simulink model "gol_cell_cl"  (R2022a)
settings: Solver=VariableStepAuto  StartTime=0.0  StopTime=10.0  RelTol=1e-3
libraries: simulink_extras x9
settings Model: Creator=SoLoMoN  LastModifiedBy=SoLoMoN

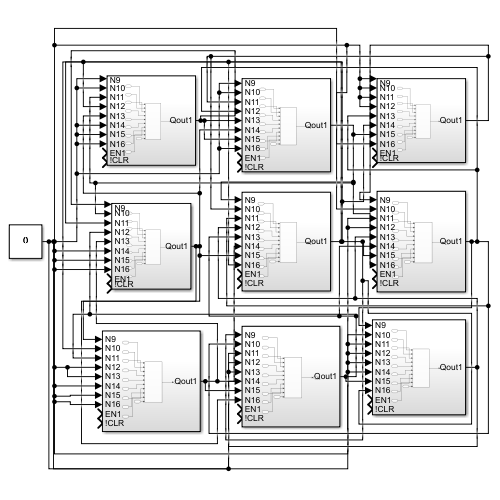
[thumbnail: Simulink's stored preview of the top-level diagram]
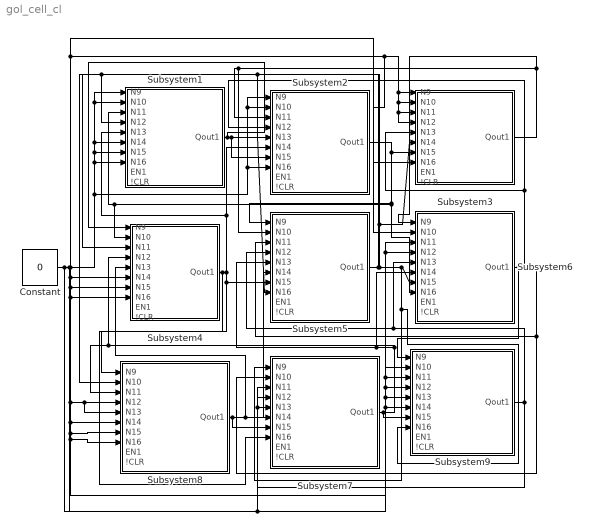
== system gol_cell_cl ==
  Constant : Constant  Value=0
  Subsystem1 : Subsystem
  Subsystem2 : Subsystem
  Subsystem3 : Subsystem
  Subsystem4 : Subsystem
  Subsystem5 : Subsystem
  Subsystem6 : Subsystem
  Subsystem7 : Subsystem
  Subsystem8 : Subsystem
  Subsystem9 : Subsystem
  wires:
  Subsystem4/1(Qout1) -> Subsystem7/8(N16), Subsystem8/1(N9), Subsystem5/7(N15), Subsystem1/5(N13), Subsystem2/6(N14)
  Subsystem2/1(Qout1) -> Subsystem6/8(N16), Subsystem4/2(N10), Subsystem1/3(N11), Subsystem5/1(N9), Subsystem3/7(N15)
  Subsystem3/1(Qout1) -> Subsystem6/1(N9), Subsystem2/3(N11), Subsystem5/2(N10)
  Subsystem6/1(Qout1) -> Subsystem7/2(N10), Subsystem5/3(N11), Subsystem3/5(N13), Subsystem2/4(N12), Subsystem9/1(N9)
  Subsystem9/1(Qout1) -> Subsystem7/3(N11), Subsystem6/5(N13), Subsystem5/4(N12)
  Subsystem7/1(Qout1) -> Subsystem9/7(N15), Subsystem8/3(N11), Subsystem4/4(N12), Subsystem6/6(N14), Subsystem5/5(N13)
  Subsystem8/1(Qout1) -> Subsystem7/7(N15), Subsystem4/5(N13), Subsystem5/6(N14)
  Subsystem1/1(Qout1) -> Subsystem4/1(N9), Subsystem2/7(N15), Subsystem5/8(N16)
  Constant/1 -> Subsystem9/6(N14), Subsystem9/3(N11), Subsystem9/2(N10), Subsystem9/4(N12), Subsystem9/5(N13), Subsystem7/6(N14), Subsystem7/5(N13), Subsystem7/4(N12), Subsystem6/2(N10), Subsystem3/4(N12), Subsystem3/3(N11), Subsystem3/2(N10), Subsystem3/1(N9), Subsystem3/8(N16), Subsystem8/5(N13), Subsystem8/4(N12), Subsystem8/6(N14), Subsystem8/7(N15), Subsystem8/8(N16), Subsystem6/4(N12), Subsystem6/3(N11), Subsystem4/8(N16), Subsystem4/7(N15), Subsystem4/6(N14), Subsystem1/7(N15), Subsystem1/6(N14), Subsystem1/2(N10), Subsystem1/1(N9), Subsystem1/8(N16), Subsystem2/8(N16), Subsystem2/2(N10), Subsystem2/1(N9)
  Subsystem5/1(Qout1) -> Subsystem9/8(N16), Subsystem7/1(N9), Subsystem6/7(N15), Subsystem4/3(N11), Subsystem1/4(N12), Subsystem2/5(N13), Subsystem3/6(N14), Subsystem8/2(N10)

== system gol_cell_cl/Subsystem1 ==
  N9 : Inport
  N10 : Inport  Port=2
  N11 : Inport  Port=3
  N12 : Inport  Port=4
  N13 : Inport  Port=5
  N14 : Inport  Port=6
  N15 : Inport  Port=7
  N16 : Inport  Port=8
  EN1 : Inport  Port=9
  !CLR : Inport  Port=10
  cell (1,1) : Subsystem
  Qout1 : Outport
  wires:
  EN1/1 -> cell (1,1)/8(EN)
  N12/1 -> cell (1,1)/4(N4)
  N13/1 -> cell (1,1)/5(N5)
  N14/1 -> cell (1,1)/6(N6)
  N15/1 -> cell (1,1)/7(N7)
  N10/1 -> cell (1,1)/2(N2)
  cell (1,1)/1(Qout) -> Qout1/1
  !CLR/1 -> cell (1,1)/10(!CLR)
  N9/1 -> cell (1,1)/1(N1)
  N11/1 -> cell (1,1)/3(N3)
  N16/1 -> cell (1,1)/9(N8)

== system gol_cell_cl/Subsystem2 ==
  N9 : Inport
  N10 : Inport  Port=2
  N11 : Inport  Port=3
  N12 : Inport  Port=4
  N13 : Inport  Port=5
  N14 : Inport  Port=6
  N15 : Inport  Port=7
  N16 : Inport  Port=8
  EN1 : Inport  Port=9
  !CLR : Inport  Port=10
  cell (1,1) : Subsystem
  Qout1 : Outport
  wires:
  EN1/1 -> cell (1,1)/8(EN)
  N12/1 -> cell (1,1)/4(N4)
  N13/1 -> cell (1,1)/5(N5)
  N14/1 -> cell (1,1)/6(N6)
  N15/1 -> cell (1,1)/7(N7)
  N10/1 -> cell (1,1)/2(N2)
  cell (1,1)/1(Qout) -> Qout1/1
  !CLR/1 -> cell (1,1)/10(!CLR)
  N9/1 -> cell (1,1)/1(N1)
  N11/1 -> cell (1,1)/3(N3)
  N16/1 -> cell (1,1)/9(N8)

== system gol_cell_cl/Subsystem3 ==
  N9 : Inport
  N10 : Inport  Port=2
  N11 : Inport  Port=3
  N12 : Inport  Port=4
  N13 : Inport  Port=5
  N14 : Inport  Port=6
  N15 : Inport  Port=7
  N16 : Inport  Port=8
  EN1 : Inport  Port=9
  !CLR : Inport  Port=10
  cell (1,1) : Subsystem
  Qout1 : Outport
  wires:
  EN1/1 -> cell (1,1)/8(EN)
  N12/1 -> cell (1,1)/4(N4)
  N13/1 -> cell (1,1)/5(N5)
  N14/1 -> cell (1,1)/6(N6)
  N15/1 -> cell (1,1)/7(N7)
  N10/1 -> cell (1,1)/2(N2)
  cell (1,1)/1(Qout) -> Qout1/1
  !CLR/1 -> cell (1,1)/10(!CLR)
  N9/1 -> cell (1,1)/1(N1)
  N11/1 -> cell (1,1)/3(N3)
  N16/1 -> cell (1,1)/9(N8)

== system gol_cell_cl/Subsystem4 ==
  N9 : Inport
  N10 : Inport  Port=2
  N11 : Inport  Port=3
  N12 : Inport  Port=4
  N13 : Inport  Port=5
  N14 : Inport  Port=6
  N15 : Inport  Port=7
  N16 : Inport  Port=8
  EN1 : Inport  Port=9
  !CLR : Inport  Port=10
  cell (1,1) : Subsystem
  Qout1 : Outport
  wires:
  EN1/1 -> cell (1,1)/8(EN)
  N12/1 -> cell (1,1)/4(N4)
  N13/1 -> cell (1,1)/5(N5)
  N14/1 -> cell (1,1)/6(N6)
  N15/1 -> cell (1,1)/7(N7)
  N10/1 -> cell (1,1)/2(N2)
  cell (1,1)/1(Qout) -> Qout1/1
  !CLR/1 -> cell (1,1)/10(!CLR)
  N9/1 -> cell (1,1)/1(N1)
  N11/1 -> cell (1,1)/3(N3)
  N16/1 -> cell (1,1)/9(N8)

== system gol_cell_cl/Subsystem5 ==
  N9 : Inport
  N10 : Inport  Port=2
  N11 : Inport  Port=3
  N12 : Inport  Port=4
  N13 : Inport  Port=5
  N14 : Inport  Port=6
  N15 : Inport  Port=7
  N16 : Inport  Port=8
  EN1 : Inport  Port=9
  !CLR : Inport  Port=10
  cell (1,1) : Subsystem
  Qout1 : Outport
  wires:
  EN1/1 -> cell (1,1)/8(EN)
  N12/1 -> cell (1,1)/4(N4)
  N13/1 -> cell (1,1)/5(N5)
  N14/1 -> cell (1,1)/6(N6)
  N15/1 -> cell (1,1)/7(N7)
  N10/1 -> cell (1,1)/2(N2)
  cell (1,1)/1(Qout) -> Qout1/1
  !CLR/1 -> cell (1,1)/10(!CLR)
  N9/1 -> cell (1,1)/1(N1)
  N11/1 -> cell (1,1)/3(N3)
  N16/1 -> cell (1,1)/9(N8)

== system gol_cell_cl/Subsystem6 ==
  N9 : Inport
  N10 : Inport  Port=2
  N11 : Inport  Port=3
  N12 : Inport  Port=4
  N13 : Inport  Port=5
  N14 : Inport  Port=6
  N15 : Inport  Port=7
  N16 : Inport  Port=8
  EN1 : Inport  Port=9
  !CLR : Inport  Port=10
  cell (1,1) : Subsystem
  Qout1 : Outport
  wires:
  EN1/1 -> cell (1,1)/8(EN)
  N12/1 -> cell (1,1)/4(N4)
  N13/1 -> cell (1,1)/5(N5)
  N14/1 -> cell (1,1)/6(N6)
  N15/1 -> cell (1,1)/7(N7)
  N10/1 -> cell (1,1)/2(N2)
  cell (1,1)/1(Qout) -> Qout1/1
  !CLR/1 -> cell (1,1)/10(!CLR)
  N9/1 -> cell (1,1)/1(N1)
  N11/1 -> cell (1,1)/3(N3)
  N16/1 -> cell (1,1)/9(N8)

== system gol_cell_cl/Subsystem7 ==
  N9 : Inport
  N10 : Inport  Port=2
  N11 : Inport  Port=3
  N12 : Inport  Port=4
  N13 : Inport  Port=5
  N14 : Inport  Port=6
  N15 : Inport  Port=7
  N16 : Inport  Port=8
  EN1 : Inport  Port=9
  !CLR : Inport  Port=10
  cell (1,1) : Subsystem
  Qout1 : Outport
  wires:
  EN1/1 -> cell (1,1)/8(EN)
  N12/1 -> cell (1,1)/4(N4)
  N13/1 -> cell (1,1)/5(N5)
  N14/1 -> cell (1,1)/6(N6)
  N15/1 -> cell (1,1)/7(N7)
  N10/1 -> cell (1,1)/2(N2)
  cell (1,1)/1(Qout) -> Qout1/1
  !CLR/1 -> cell (1,1)/10(!CLR)
  N9/1 -> cell (1,1)/1(N1)
  N11/1 -> cell (1,1)/3(N3)
  N16/1 -> cell (1,1)/9(N8)

== system gol_cell_cl/Subsystem8 ==
  N9 : Inport
  N10 : Inport  Port=2
  N11 : Inport  Port=3
  N12 : Inport  Port=4
  N13 : Inport  Port=5
  N14 : Inport  Port=6
  N15 : Inport  Port=7
  N16 : Inport  Port=8
  EN1 : Inport  Port=9
  !CLR : Inport  Port=10
  cell (1,1) : Subsystem
  Qout1 : Outport
  wires:
  EN1/1 -> cell (1,1)/8(EN)
  N12/1 -> cell (1,1)/4(N4)
  N13/1 -> cell (1,1)/5(N5)
  N14/1 -> cell (1,1)/6(N6)
  N15/1 -> cell (1,1)/7(N7)
  N10/1 -> cell (1,1)/2(N2)
  cell (1,1)/1(Qout) -> Qout1/1
  !CLR/1 -> cell (1,1)/10(!CLR)
  N9/1 -> cell (1,1)/1(N1)
  N11/1 -> cell (1,1)/3(N3)
  N16/1 -> cell (1,1)/9(N8)

== system gol_cell_cl/Subsystem9 ==
  N9 : Inport
  N10 : Inport  Port=2
  N11 : Inport  Port=3
  N12 : Inport  Port=4
  N13 : Inport  Port=5
  N14 : Inport  Port=6
  N15 : Inport  Port=7
  N16 : Inport  Port=8
  EN1 : Inport  Port=9
  !CLR : Inport  Port=10
  cell (1,1) : Subsystem
  Qout1 : Outport
  wires:
  EN1/1 -> cell (1,1)/8(EN)
  N12/1 -> cell (1,1)/4(N4)
  N13/1 -> cell (1,1)/5(N5)
  N14/1 -> cell (1,1)/6(N6)
  N15/1 -> cell (1,1)/7(N7)
  N10/1 -> cell (1,1)/2(N2)
  cell (1,1)/1(Qout) -> Qout1/1
  !CLR/1 -> cell (1,1)/10(!CLR)
  N9/1 -> cell (1,1)/1(N1)
  N11/1 -> cell (1,1)/3(N3)
  N16/1 -> cell (1,1)/9(N8)

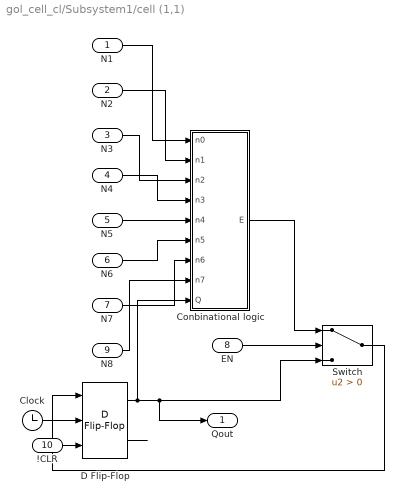
== system gol_cell_cl/Subsystem1/cell (1,1) ==
  N1 : Inport
  N2 : Inport  Port=2
  N3 : Inport  Port=3
  N4 : Inport  Port=4
  N5 : Inport  Port=5
  N6 : Inport  Port=6
  N7 : Inport  Port=7
  EN : Inport  Port=8
  N8 : Inport  Port=9
  !CLR : Inport  Port=10
  Clock : Clock
  Conbinational logic : Subsystem
  D Flip-Flop : simulink_extras/Flip Flops/D Flip-Flop
  Switch : Switch  Criteria=u2 > Threshold  SaturateOnIntegerOverflow=off  InputSameDT=off
  Qout : Outport
  wires:
  N3/1 -> Conbinational logic/3(n2)
  N1/1 -> Conbinational logic/1(n0)
  Clock/1 -> D Flip-Flop/2
  Conbinational logic/1(E) -> Switch/1
  Switch/1 -> D Flip-Flop/1
  D Flip-Flop/1 -> Qout/1, Switch/3, Conbinational logic/9(Q)
  N6/1 -> Conbinational logic/6(n5)
  EN/1 -> Switch/2
  N2/1 -> Conbinational logic/2(n1)
  N7/1 -> Conbinational logic/7(n6)
  N4/1 -> Conbinational logic/4(n3)
  N5/1 -> Conbinational logic/5(n4)
  N8/1 -> Conbinational logic/8(n7)
  !CLR/1 -> D Flip-Flop/3
  D Flip-Flop/2 -> ?

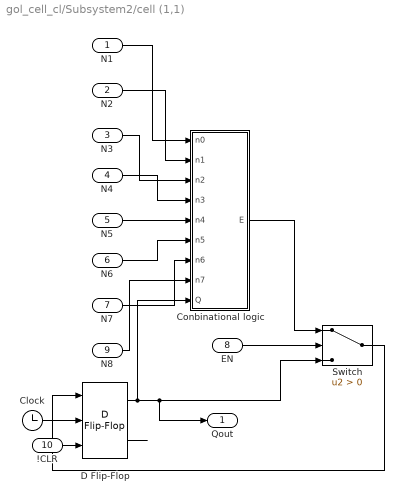
== system gol_cell_cl/Subsystem2/cell (1,1) ==
  N1 : Inport
  N2 : Inport  Port=2
  N3 : Inport  Port=3
  N4 : Inport  Port=4
  N5 : Inport  Port=5
  N6 : Inport  Port=6
  N7 : Inport  Port=7
  EN : Inport  Port=8
  N8 : Inport  Port=9
  !CLR : Inport  Port=10
  Clock : Clock
  Conbinational logic : Subsystem
  D Flip-Flop : simulink_extras/Flip Flops/D Flip-Flop
  Switch : Switch  Criteria=u2 > Threshold  SaturateOnIntegerOverflow=off  InputSameDT=off
  Qout : Outport
  wires:
  N3/1 -> Conbinational logic/3(n2)
  N1/1 -> Conbinational logic/1(n0)
  Clock/1 -> D Flip-Flop/2
  Conbinational logic/1(E) -> Switch/1
  Switch/1 -> D Flip-Flop/1
  D Flip-Flop/1 -> Qout/1, Switch/3, Conbinational logic/9(Q)
  N6/1 -> Conbinational logic/6(n5)
  EN/1 -> Switch/2
  N2/1 -> Conbinational logic/2(n1)
  N7/1 -> Conbinational logic/7(n6)
  N4/1 -> Conbinational logic/4(n3)
  N5/1 -> Conbinational logic/5(n4)
  N8/1 -> Conbinational logic/8(n7)
  !CLR/1 -> D Flip-Flop/3
  D Flip-Flop/2 -> ?

== system gol_cell_cl/Subsystem3/cell (1,1) ==
  N1 : Inport
  N2 : Inport  Port=2
  N3 : Inport  Port=3
  N4 : Inport  Port=4
  N5 : Inport  Port=5
  N6 : Inport  Port=6
  N7 : Inport  Port=7
  EN : Inport  Port=8
  N8 : Inport  Port=9
  !CLR : Inport  Port=10
  Clock : Clock
  Conbinational logic : Subsystem
  D Flip-Flop : simulink_extras/Flip Flops/D Flip-Flop
  Switch : Switch  Criteria=u2 > Threshold  SaturateOnIntegerOverflow=off  InputSameDT=off
  Qout : Outport
  wires:
  N3/1 -> Conbinational logic/3(n2)
  N1/1 -> Conbinational logic/1(n0)
  Clock/1 -> D Flip-Flop/2
  Conbinational logic/1(E) -> Switch/1
  Switch/1 -> D Flip-Flop/1
  D Flip-Flop/1 -> Qout/1, Switch/3, Conbinational logic/9(Q)
  N6/1 -> Conbinational logic/6(n5)
  EN/1 -> Switch/2
  N2/1 -> Conbinational logic/2(n1)
  N7/1 -> Conbinational logic/7(n6)
  N4/1 -> Conbinational logic/4(n3)
  N5/1 -> Conbinational logic/5(n4)
  N8/1 -> Conbinational logic/8(n7)
  !CLR/1 -> D Flip-Flop/3
  D Flip-Flop/2 -> ?

== system gol_cell_cl/Subsystem4/cell (1,1) ==
  N1 : Inport
  N2 : Inport  Port=2
  N3 : Inport  Port=3
  N4 : Inport  Port=4
  N5 : Inport  Port=5
  N6 : Inport  Port=6
  N7 : Inport  Port=7
  EN : Inport  Port=8
  N8 : Inport  Port=9
  !CLR : Inport  Port=10
  Clock : Clock
  Conbinational logic : Subsystem
  D Flip-Flop : simulink_extras/Flip Flops/D Flip-Flop
  Switch : Switch  Criteria=u2 > Threshold  SaturateOnIntegerOverflow=off  InputSameDT=off
  Qout : Outport
  wires:
  N3/1 -> Conbinational logic/3(n2)
  N1/1 -> Conbinational logic/1(n0)
  Clock/1 -> D Flip-Flop/2
  Conbinational logic/1(E) -> Switch/1
  Switch/1 -> D Flip-Flop/1
  D Flip-Flop/1 -> Qout/1, Switch/3, Conbinational logic/9(Q)
  N6/1 -> Conbinational logic/6(n5)
  EN/1 -> Switch/2
  N2/1 -> Conbinational logic/2(n1)
  N7/1 -> Conbinational logic/7(n6)
  N4/1 -> Conbinational logic/4(n3)
  N5/1 -> Conbinational logic/5(n4)
  N8/1 -> Conbinational logic/8(n7)
  !CLR/1 -> D Flip-Flop/3
  D Flip-Flop/2 -> ?

== system gol_cell_cl/Subsystem5/cell (1,1) ==
  N1 : Inport
  N2 : Inport  Port=2
  N3 : Inport  Port=3
  N4 : Inport  Port=4
  N5 : Inport  Port=5
  N6 : Inport  Port=6
  N7 : Inport  Port=7
  EN : Inport  Port=8
  N8 : Inport  Port=9
  !CLR : Inport  Port=10
  Clock : Clock
  Conbinational logic : Subsystem
  D Flip-Flop : simulink_extras/Flip Flops/D Flip-Flop
  Switch : Switch  Criteria=u2 > Threshold  SaturateOnIntegerOverflow=off  InputSameDT=off
  Qout : Outport
  wires:
  N3/1 -> Conbinational logic/3(n2)
  N1/1 -> Conbinational logic/1(n0)
  Clock/1 -> D Flip-Flop/2
  Conbinational logic/1(E) -> Switch/1
  Switch/1 -> D Flip-Flop/1
  D Flip-Flop/1 -> Qout/1, Switch/3, Conbinational logic/9(Q)
  N6/1 -> Conbinational logic/6(n5)
  EN/1 -> Switch/2
  N2/1 -> Conbinational logic/2(n1)
  N7/1 -> Conbinational logic/7(n6)
  N4/1 -> Conbinational logic/4(n3)
  N5/1 -> Conbinational logic/5(n4)
  N8/1 -> Conbinational logic/8(n7)
  !CLR/1 -> D Flip-Flop/3
  D Flip-Flop/2 -> ?

== system gol_cell_cl/Subsystem6/cell (1,1) ==
  N1 : Inport
  N2 : Inport  Port=2
  N3 : Inport  Port=3
  N4 : Inport  Port=4
  N5 : Inport  Port=5
  N6 : Inport  Port=6
  N7 : Inport  Port=7
  EN : Inport  Port=8
  N8 : Inport  Port=9
  !CLR : Inport  Port=10
  Clock : Clock
  Conbinational logic : Subsystem
  D Flip-Flop : simulink_extras/Flip Flops/D Flip-Flop
  Switch : Switch  Criteria=u2 > Threshold  SaturateOnIntegerOverflow=off  InputSameDT=off
  Qout : Outport
  wires:
  N3/1 -> Conbinational logic/3(n2)
  N1/1 -> Conbinational logic/1(n0)
  Clock/1 -> D Flip-Flop/2
  Conbinational logic/1(E) -> Switch/1
  Switch/1 -> D Flip-Flop/1
  D Flip-Flop/1 -> Qout/1, Switch/3, Conbinational logic/9(Q)
  N6/1 -> Conbinational logic/6(n5)
  EN/1 -> Switch/2
  N2/1 -> Conbinational logic/2(n1)
  N7/1 -> Conbinational logic/7(n6)
  N4/1 -> Conbinational logic/4(n3)
  N5/1 -> Conbinational logic/5(n4)
  N8/1 -> Conbinational logic/8(n7)
  !CLR/1 -> D Flip-Flop/3
  D Flip-Flop/2 -> ?

== system gol_cell_cl/Subsystem7/cell (1,1) ==
  N1 : Inport
  N2 : Inport  Port=2
  N3 : Inport  Port=3
  N4 : Inport  Port=4
  N5 : Inport  Port=5
  N6 : Inport  Port=6
  N7 : Inport  Port=7
  EN : Inport  Port=8
  N8 : Inport  Port=9
  !CLR : Inport  Port=10
  Clock : Clock
  Conbinational logic : Subsystem
  D Flip-Flop : simulink_extras/Flip Flops/D Flip-Flop
  Switch : Switch  Criteria=u2 > Threshold  SaturateOnIntegerOverflow=off  InputSameDT=off
  Qout : Outport
  wires:
  N3/1 -> Conbinational logic/3(n2)
  N1/1 -> Conbinational logic/1(n0)
  Clock/1 -> D Flip-Flop/2
  Conbinational logic/1(E) -> Switch/1
  Switch/1 -> D Flip-Flop/1
  D Flip-Flop/1 -> Qout/1, Switch/3, Conbinational logic/9(Q)
  N6/1 -> Conbinational logic/6(n5)
  EN/1 -> Switch/2
  N2/1 -> Conbinational logic/2(n1)
  N7/1 -> Conbinational logic/7(n6)
  N4/1 -> Conbinational logic/4(n3)
  N5/1 -> Conbinational logic/5(n4)
  N8/1 -> Conbinational logic/8(n7)
  !CLR/1 -> D Flip-Flop/3
  D Flip-Flop/2 -> ?

== system gol_cell_cl/Subsystem8/cell (1,1) ==
  N1 : Inport
  N2 : Inport  Port=2
  N3 : Inport  Port=3
  N4 : Inport  Port=4
  N5 : Inport  Port=5
  N6 : Inport  Port=6
  N7 : Inport  Port=7
  EN : Inport  Port=8
  N8 : Inport  Port=9
  !CLR : Inport  Port=10
  Clock : Clock
  Conbinational logic : Subsystem
  D Flip-Flop : simulink_extras/Flip Flops/D Flip-Flop
  Switch : Switch  Criteria=u2 > Threshold  SaturateOnIntegerOverflow=off  InputSameDT=off
  Qout : Outport
  wires:
  N3/1 -> Conbinational logic/3(n2)
  N1/1 -> Conbinational logic/1(n0)
  Clock/1 -> D Flip-Flop/2
  Conbinational logic/1(E) -> Switch/1
  Switch/1 -> D Flip-Flop/1
  D Flip-Flop/1 -> Qout/1, Switch/3, Conbinational logic/9(Q)
  N6/1 -> Conbinational logic/6(n5)
  EN/1 -> Switch/2
  N2/1 -> Conbinational logic/2(n1)
  N7/1 -> Conbinational logic/7(n6)
  N4/1 -> Conbinational logic/4(n3)
  N5/1 -> Conbinational logic/5(n4)
  N8/1 -> Conbinational logic/8(n7)
  !CLR/1 -> D Flip-Flop/3
  D Flip-Flop/2 -> ?

== system gol_cell_cl/Subsystem9/cell (1,1) ==
  N1 : Inport
  N2 : Inport  Port=2
  N3 : Inport  Port=3
  N4 : Inport  Port=4
  N5 : Inport  Port=5
  N6 : Inport  Port=6
  N7 : Inport  Port=7
  EN : Inport  Port=8
  N8 : Inport  Port=9
  !CLR : Inport  Port=10
  Clock : Clock
  Conbinational logic : Subsystem
  D Flip-Flop : simulink_extras/Flip Flops/D Flip-Flop
  Switch : Switch  Criteria=u2 > Threshold  SaturateOnIntegerOverflow=off  InputSameDT=off
  Qout : Outport
  wires:
  N3/1 -> Conbinational logic/3(n2)
  N1/1 -> Conbinational logic/1(n0)
  Clock/1 -> D Flip-Flop/2
  Conbinational logic/1(E) -> Switch/1
  Switch/1 -> D Flip-Flop/1
  D Flip-Flop/1 -> Qout/1, Switch/3, Conbinational logic/9(Q)
  N6/1 -> Conbinational logic/6(n5)
  EN/1 -> Switch/2
  N2/1 -> Conbinational logic/2(n1)
  N7/1 -> Conbinational logic/7(n6)
  N4/1 -> Conbinational logic/4(n3)
  N5/1 -> Conbinational logic/5(n4)
  N8/1 -> Conbinational logic/8(n7)
  !CLR/1 -> D Flip-Flop/3
  D Flip-Flop/2 -> ?

== system gol_cell_cl/Subsystem1/cell (1,1)/Conbinational logic ==
  n0 : Inport
  n1 : Inport  Port=2
  n2 : Inport  Port=3
  n3 : Inport  Port=4
  n4 : Inport  Port=5
  n5 : Inport  Port=6
  n6 : Inport  Port=7
  n7 : Inport  Port=8
  Q : Inport  Port=9
  PACK : Subsystem
  E : Outport
  wires:
  n0/1 -> PACK/1(n0)
  n1/1 -> PACK/2(n1)
  n2/1 -> PACK/3(n2)
  n3/1 -> PACK/4(n3)
  n4/1 -> PACK/5(n4)
  n5/1 -> PACK/6(n5)
  n6/1 -> PACK/7(n6)
  n7/1 -> PACK/8(n7)
  Q/1 -> PACK/9(Q)
  PACK/1(E) -> E/1

== system gol_cell_cl/Subsystem2/cell (1,1)/Conbinational logic ==
  n0 : Inport
  n1 : Inport  Port=2
  n2 : Inport  Port=3
  n3 : Inport  Port=4
  n4 : Inport  Port=5
  n5 : Inport  Port=6
  n6 : Inport  Port=7
  n7 : Inport  Port=8
  Q : Inport  Port=9
  PACK : Subsystem
  E : Outport
  wires:
  n0/1 -> PACK/1(n0)
  n1/1 -> PACK/2(n1)
  n2/1 -> PACK/3(n2)
  n3/1 -> PACK/4(n3)
  n4/1 -> PACK/5(n4)
  n5/1 -> PACK/6(n5)
  n6/1 -> PACK/7(n6)
  n7/1 -> PACK/8(n7)
  Q/1 -> PACK/9(Q)
  PACK/1(E) -> E/1

== system gol_cell_cl/Subsystem3/cell (1,1)/Conbinational logic ==
  n0 : Inport
  n1 : Inport  Port=2
  n2 : Inport  Port=3
  n3 : Inport  Port=4
  n4 : Inport  Port=5
  n5 : Inport  Port=6
  n6 : Inport  Port=7
  n7 : Inport  Port=8
  Q : Inport  Port=9
  PACK : Subsystem
  E : Outport
  wires:
  n0/1 -> PACK/1(n0)
  n1/1 -> PACK/2(n1)
  n2/1 -> PACK/3(n2)
  n3/1 -> PACK/4(n3)
  n4/1 -> PACK/5(n4)
  n5/1 -> PACK/6(n5)
  n6/1 -> PACK/7(n6)
  n7/1 -> PACK/8(n7)
  Q/1 -> PACK/9(Q)
  PACK/1(E) -> E/1

== system gol_cell_cl/Subsystem4/cell (1,1)/Conbinational logic ==
  n0 : Inport
  n1 : Inport  Port=2
  n2 : Inport  Port=3
  n3 : Inport  Port=4
  n4 : Inport  Port=5
  n5 : Inport  Port=6
  n6 : Inport  Port=7
  n7 : Inport  Port=8
  Q : Inport  Port=9
  PACK : Subsystem
  E : Outport
  wires:
  n0/1 -> PACK/1(n0)
  n1/1 -> PACK/2(n1)
  n2/1 -> PACK/3(n2)
  n3/1 -> PACK/4(n3)
  n4/1 -> PACK/5(n4)
  n5/1 -> PACK/6(n5)
  n6/1 -> PACK/7(n6)
  n7/1 -> PACK/8(n7)
  Q/1 -> PACK/9(Q)
  PACK/1(E) -> E/1

== system gol_cell_cl/Subsystem5/cell (1,1)/Conbinational logic ==
  n0 : Inport
  n1 : Inport  Port=2
  n2 : Inport  Port=3
  n3 : Inport  Port=4
  n4 : Inport  Port=5
  n5 : Inport  Port=6
  n6 : Inport  Port=7
  n7 : Inport  Port=8
  Q : Inport  Port=9
  PACK : Subsystem
  E : Outport
  wires:
  n0/1 -> PACK/1(n0)
  n1/1 -> PACK/2(n1)
  n2/1 -> PACK/3(n2)
  n3/1 -> PACK/4(n3)
  n4/1 -> PACK/5(n4)
  n5/1 -> PACK/6(n5)
  n6/1 -> PACK/7(n6)
  n7/1 -> PACK/8(n7)
  Q/1 -> PACK/9(Q)
  PACK/1(E) -> E/1

== system gol_cell_cl/Subsystem6/cell (1,1)/Conbinational logic ==
  n0 : Inport
  n1 : Inport  Port=2
  n2 : Inport  Port=3
  n3 : Inport  Port=4
  n4 : Inport  Port=5
  n5 : Inport  Port=6
  n6 : Inport  Port=7
  n7 : Inport  Port=8
  Q : Inport  Port=9
  PACK : Subsystem
  E : Outport
  wires:
  n0/1 -> PACK/1(n0)
  n1/1 -> PACK/2(n1)
  n2/1 -> PACK/3(n2)
  n3/1 -> PACK/4(n3)
  n4/1 -> PACK/5(n4)
  n5/1 -> PACK/6(n5)
  n6/1 -> PACK/7(n6)
  n7/1 -> PACK/8(n7)
  Q/1 -> PACK/9(Q)
  PACK/1(E) -> E/1

== system gol_cell_cl/Subsystem7/cell (1,1)/Conbinational logic ==
  n0 : Inport
  n1 : Inport  Port=2
  n2 : Inport  Port=3
  n3 : Inport  Port=4
  n4 : Inport  Port=5
  n5 : Inport  Port=6
  n6 : Inport  Port=7
  n7 : Inport  Port=8
  Q : Inport  Port=9
  PACK : Subsystem
  E : Outport
  wires:
  n0/1 -> PACK/1(n0)
  n1/1 -> PACK/2(n1)
  n2/1 -> PACK/3(n2)
  n3/1 -> PACK/4(n3)
  n4/1 -> PACK/5(n4)
  n5/1 -> PACK/6(n5)
  n6/1 -> PACK/7(n6)
  n7/1 -> PACK/8(n7)
  Q/1 -> PACK/9(Q)
  PACK/1(E) -> E/1

== system gol_cell_cl/Subsystem8/cell (1,1)/Conbinational logic ==
  n0 : Inport
  n1 : Inport  Port=2
  n2 : Inport  Port=3
  n3 : Inport  Port=4
  n4 : Inport  Port=5
  n5 : Inport  Port=6
  n6 : Inport  Port=7
  n7 : Inport  Port=8
  Q : Inport  Port=9
  PACK : Subsystem
  E : Outport
  wires:
  n0/1 -> PACK/1(n0)
  n1/1 -> PACK/2(n1)
  n2/1 -> PACK/3(n2)
  n3/1 -> PACK/4(n3)
  n4/1 -> PACK/5(n4)
  n5/1 -> PACK/6(n5)
  n6/1 -> PACK/7(n6)
  n7/1 -> PACK/8(n7)
  Q/1 -> PACK/9(Q)
  PACK/1(E) -> E/1

== system gol_cell_cl/Subsystem9/cell (1,1)/Conbinational logic ==
  n0 : Inport
  n1 : Inport  Port=2
  n2 : Inport  Port=3
  n3 : Inport  Port=4
  n4 : Inport  Port=5
  n5 : Inport  Port=6
  n6 : Inport  Port=7
  n7 : Inport  Port=8
  Q : Inport  Port=9
  PACK : Subsystem
  E : Outport
  wires:
  n0/1 -> PACK/1(n0)
  n1/1 -> PACK/2(n1)
  n2/1 -> PACK/3(n2)
  n3/1 -> PACK/4(n3)
  n4/1 -> PACK/5(n4)
  n5/1 -> PACK/6(n5)
  n6/1 -> PACK/7(n6)
  n7/1 -> PACK/8(n7)
  Q/1 -> PACK/9(Q)
  PACK/1(E) -> E/1

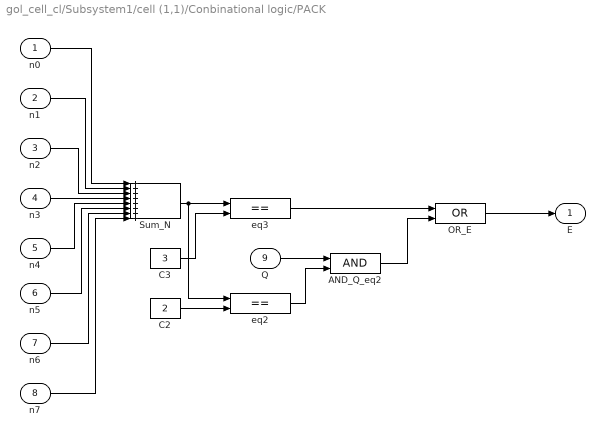
== system gol_cell_cl/Subsystem1/cell (1,1)/Conbinational logic/PACK ==
  n0 : Inport
  n1 : Inport  Port=2
  n2 : Inport  Port=3
  n3 : Inport  Port=4
  n4 : Inport  Port=5
  n5 : Inport  Port=6
  n6 : Inport  Port=7
  n7 : Inport  Port=8
  Q : Inport  Port=9
  AND_Q_eq2 : Logic  AllPortsSameDT=off  OutDataTypeStr=boolean
  C2 : Constant  Value=2  OutDataTypeStr=fixdt(0,4,0)
  C3 : Constant  Value=3  OutDataTypeStr=fixdt(0,4,0)
  OR_E : Logic  Operator=OR  AllPortsSameDT=off  OutDataTypeStr=boolean
  Sum_N : Sum  Inputs=++++++++  AccumDataTypeStr=fixdt(0,4,0)  OutDataTypeStr=fixdt(0,4,0)
  eq2 : RelationalOperator  Operator===  OutDataTypeStr=boolean  RndMeth=Simplest  InputSameDT=off
  eq3 : RelationalOperator  Operator===  OutDataTypeStr=boolean  RndMeth=Simplest  InputSameDT=off
  E : Outport
  wires:
  Sum_N/1 -> eq2/1, eq3/1
  C3/1 -> eq3/2
  n7/1 -> Sum_N/8
  Q/1 -> AND_Q_eq2/1
  n0/1 -> Sum_N/1
  n3/1 -> Sum_N/4
  eq3/1 -> OR_E/1
  n1/1 -> Sum_N/2
  n4/1 -> Sum_N/5
  n2/1 -> Sum_N/3
  n6/1 -> Sum_N/7
  eq2/1 -> AND_Q_eq2/2
  C2/1 -> eq2/2
  OR_E/1 -> E/1
  AND_Q_eq2/1 -> OR_E/2
  n5/1 -> Sum_N/6

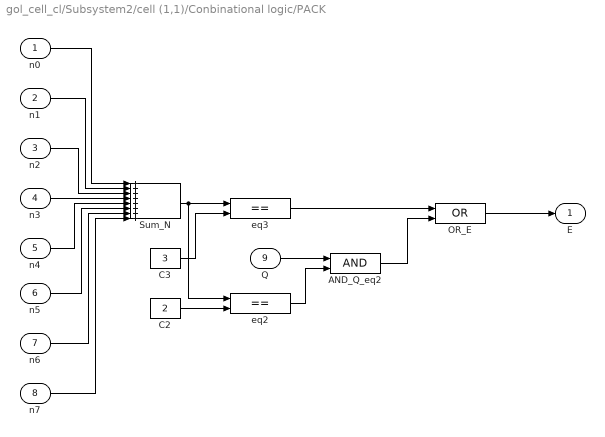
== system gol_cell_cl/Subsystem2/cell (1,1)/Conbinational logic/PACK ==
  n0 : Inport
  n1 : Inport  Port=2
  n2 : Inport  Port=3
  n3 : Inport  Port=4
  n4 : Inport  Port=5
  n5 : Inport  Port=6
  n6 : Inport  Port=7
  n7 : Inport  Port=8
  Q : Inport  Port=9
  AND_Q_eq2 : Logic  AllPortsSameDT=off  OutDataTypeStr=boolean
  C2 : Constant  Value=2  OutDataTypeStr=fixdt(0,4,0)
  C3 : Constant  Value=3  OutDataTypeStr=fixdt(0,4,0)
  OR_E : Logic  Operator=OR  AllPortsSameDT=off  OutDataTypeStr=boolean
  Sum_N : Sum  Inputs=++++++++  AccumDataTypeStr=fixdt(0,4,0)  OutDataTypeStr=fixdt(0,4,0)
  eq2 : RelationalOperator  Operator===  OutDataTypeStr=boolean  RndMeth=Simplest  InputSameDT=off
  eq3 : RelationalOperator  Operator===  OutDataTypeStr=boolean  RndMeth=Simplest  InputSameDT=off
  E : Outport
  wires:
  Sum_N/1 -> eq2/1, eq3/1
  C3/1 -> eq3/2
  n7/1 -> Sum_N/8
  Q/1 -> AND_Q_eq2/1
  n0/1 -> Sum_N/1
  n3/1 -> Sum_N/4
  eq3/1 -> OR_E/1
  n1/1 -> Sum_N/2
  n4/1 -> Sum_N/5
  n2/1 -> Sum_N/3
  n6/1 -> Sum_N/7
  eq2/1 -> AND_Q_eq2/2
  C2/1 -> eq2/2
  OR_E/1 -> E/1
  AND_Q_eq2/1 -> OR_E/2
  n5/1 -> Sum_N/6

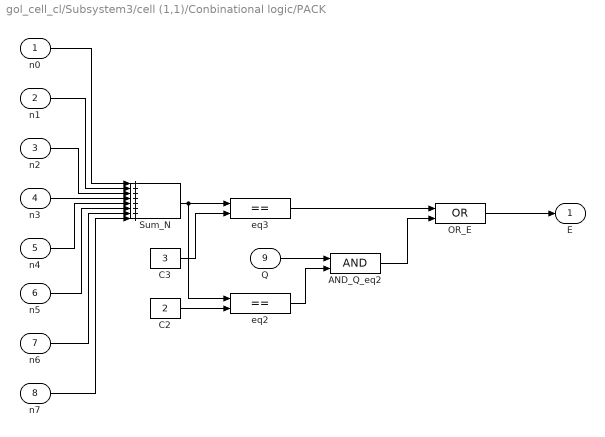
== system gol_cell_cl/Subsystem3/cell (1,1)/Conbinational logic/PACK ==
  n0 : Inport
  n1 : Inport  Port=2
  n2 : Inport  Port=3
  n3 : Inport  Port=4
  n4 : Inport  Port=5
  n5 : Inport  Port=6
  n6 : Inport  Port=7
  n7 : Inport  Port=8
  Q : Inport  Port=9
  AND_Q_eq2 : Logic  AllPortsSameDT=off  OutDataTypeStr=boolean
  C2 : Constant  Value=2  OutDataTypeStr=fixdt(0,4,0)
  C3 : Constant  Value=3  OutDataTypeStr=fixdt(0,4,0)
  OR_E : Logic  Operator=OR  AllPortsSameDT=off  OutDataTypeStr=boolean
  Sum_N : Sum  Inputs=++++++++  AccumDataTypeStr=fixdt(0,4,0)  OutDataTypeStr=fixdt(0,4,0)
  eq2 : RelationalOperator  Operator===  OutDataTypeStr=boolean  RndMeth=Simplest  InputSameDT=off
  eq3 : RelationalOperator  Operator===  OutDataTypeStr=boolean  RndMeth=Simplest  InputSameDT=off
  E : Outport
  wires:
  Sum_N/1 -> eq2/1, eq3/1
  C3/1 -> eq3/2
  n7/1 -> Sum_N/8
  Q/1 -> AND_Q_eq2/1
  n0/1 -> Sum_N/1
  n3/1 -> Sum_N/4
  eq3/1 -> OR_E/1
  n1/1 -> Sum_N/2
  n4/1 -> Sum_N/5
  n2/1 -> Sum_N/3
  n6/1 -> Sum_N/7
  eq2/1 -> AND_Q_eq2/2
  C2/1 -> eq2/2
  OR_E/1 -> E/1
  AND_Q_eq2/1 -> OR_E/2
  n5/1 -> Sum_N/6

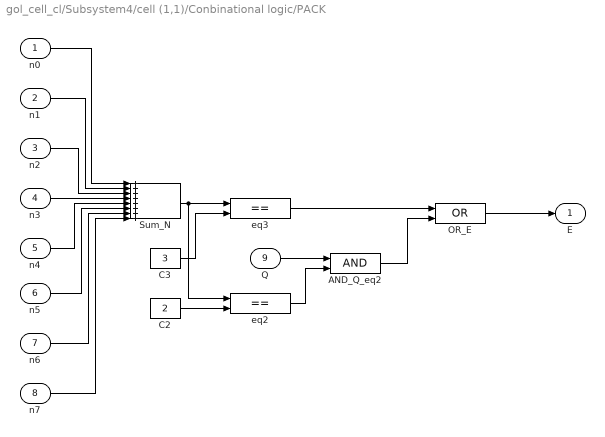
== system gol_cell_cl/Subsystem4/cell (1,1)/Conbinational logic/PACK ==
  n0 : Inport
  n1 : Inport  Port=2
  n2 : Inport  Port=3
  n3 : Inport  Port=4
  n4 : Inport  Port=5
  n5 : Inport  Port=6
  n6 : Inport  Port=7
  n7 : Inport  Port=8
  Q : Inport  Port=9
  AND_Q_eq2 : Logic  AllPortsSameDT=off  OutDataTypeStr=boolean
  C2 : Constant  Value=2  OutDataTypeStr=fixdt(0,4,0)
  C3 : Constant  Value=3  OutDataTypeStr=fixdt(0,4,0)
  OR_E : Logic  Operator=OR  AllPortsSameDT=off  OutDataTypeStr=boolean
  Sum_N : Sum  Inputs=++++++++  AccumDataTypeStr=fixdt(0,4,0)  OutDataTypeStr=fixdt(0,4,0)
  eq2 : RelationalOperator  Operator===  OutDataTypeStr=boolean  RndMeth=Simplest  InputSameDT=off
  eq3 : RelationalOperator  Operator===  OutDataTypeStr=boolean  RndMeth=Simplest  InputSameDT=off
  E : Outport
  wires:
  Sum_N/1 -> eq2/1, eq3/1
  C3/1 -> eq3/2
  n7/1 -> Sum_N/8
  Q/1 -> AND_Q_eq2/1
  n0/1 -> Sum_N/1
  n3/1 -> Sum_N/4
  eq3/1 -> OR_E/1
  n1/1 -> Sum_N/2
  n4/1 -> Sum_N/5
  n2/1 -> Sum_N/3
  n6/1 -> Sum_N/7
  eq2/1 -> AND_Q_eq2/2
  C2/1 -> eq2/2
  OR_E/1 -> E/1
  AND_Q_eq2/1 -> OR_E/2
  n5/1 -> Sum_N/6

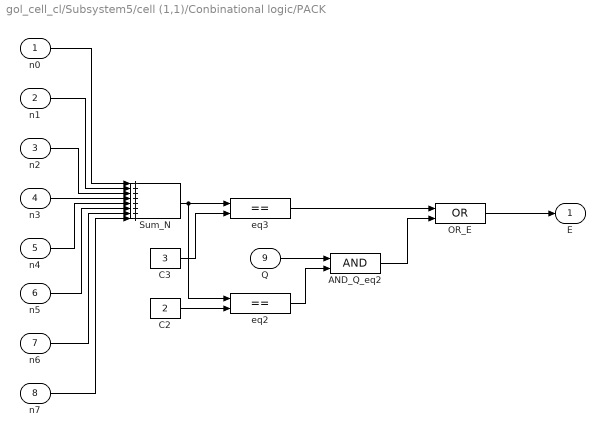
== system gol_cell_cl/Subsystem5/cell (1,1)/Conbinational logic/PACK ==
  n0 : Inport
  n1 : Inport  Port=2
  n2 : Inport  Port=3
  n3 : Inport  Port=4
  n4 : Inport  Port=5
  n5 : Inport  Port=6
  n6 : Inport  Port=7
  n7 : Inport  Port=8
  Q : Inport  Port=9
  AND_Q_eq2 : Logic  AllPortsSameDT=off  OutDataTypeStr=boolean
  C2 : Constant  Value=2  OutDataTypeStr=fixdt(0,4,0)
  C3 : Constant  Value=3  OutDataTypeStr=fixdt(0,4,0)
  OR_E : Logic  Operator=OR  AllPortsSameDT=off  OutDataTypeStr=boolean
  Sum_N : Sum  Inputs=++++++++  AccumDataTypeStr=fixdt(0,4,0)  OutDataTypeStr=fixdt(0,4,0)
  eq2 : RelationalOperator  Operator===  OutDataTypeStr=boolean  RndMeth=Simplest  InputSameDT=off
  eq3 : RelationalOperator  Operator===  OutDataTypeStr=boolean  RndMeth=Simplest  InputSameDT=off
  E : Outport
  wires:
  Sum_N/1 -> eq2/1, eq3/1
  C3/1 -> eq3/2
  n7/1 -> Sum_N/8
  Q/1 -> AND_Q_eq2/1
  n0/1 -> Sum_N/1
  n3/1 -> Sum_N/4
  eq3/1 -> OR_E/1
  n1/1 -> Sum_N/2
  n4/1 -> Sum_N/5
  n2/1 -> Sum_N/3
  n6/1 -> Sum_N/7
  eq2/1 -> AND_Q_eq2/2
  C2/1 -> eq2/2
  OR_E/1 -> E/1
  AND_Q_eq2/1 -> OR_E/2
  n5/1 -> Sum_N/6

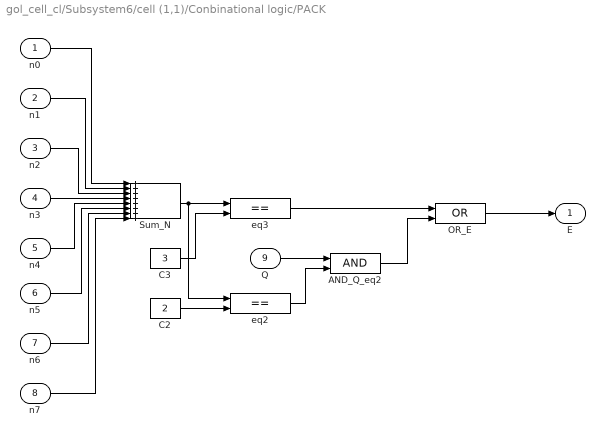
== system gol_cell_cl/Subsystem6/cell (1,1)/Conbinational logic/PACK ==
  n0 : Inport
  n1 : Inport  Port=2
  n2 : Inport  Port=3
  n3 : Inport  Port=4
  n4 : Inport  Port=5
  n5 : Inport  Port=6
  n6 : Inport  Port=7
  n7 : Inport  Port=8
  Q : Inport  Port=9
  AND_Q_eq2 : Logic  AllPortsSameDT=off  OutDataTypeStr=boolean
  C2 : Constant  Value=2  OutDataTypeStr=fixdt(0,4,0)
  C3 : Constant  Value=3  OutDataTypeStr=fixdt(0,4,0)
  OR_E : Logic  Operator=OR  AllPortsSameDT=off  OutDataTypeStr=boolean
  Sum_N : Sum  Inputs=++++++++  AccumDataTypeStr=fixdt(0,4,0)  OutDataTypeStr=fixdt(0,4,0)
  eq2 : RelationalOperator  Operator===  OutDataTypeStr=boolean  RndMeth=Simplest  InputSameDT=off
  eq3 : RelationalOperator  Operator===  OutDataTypeStr=boolean  RndMeth=Simplest  InputSameDT=off
  E : Outport
  wires:
  Sum_N/1 -> eq2/1, eq3/1
  C3/1 -> eq3/2
  n7/1 -> Sum_N/8
  Q/1 -> AND_Q_eq2/1
  n0/1 -> Sum_N/1
  n3/1 -> Sum_N/4
  eq3/1 -> OR_E/1
  n1/1 -> Sum_N/2
  n4/1 -> Sum_N/5
  n2/1 -> Sum_N/3
  n6/1 -> Sum_N/7
  eq2/1 -> AND_Q_eq2/2
  C2/1 -> eq2/2
  OR_E/1 -> E/1
  AND_Q_eq2/1 -> OR_E/2
  n5/1 -> Sum_N/6

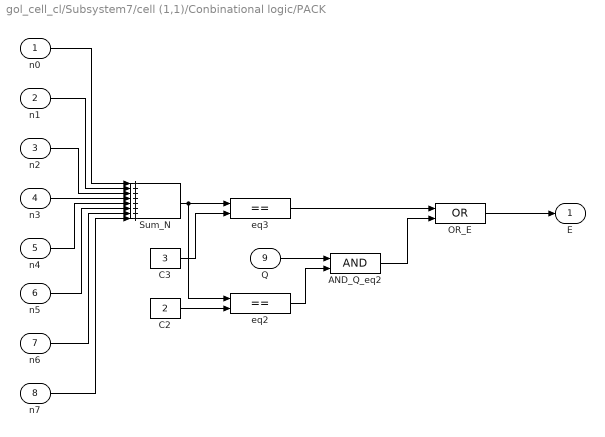
== system gol_cell_cl/Subsystem7/cell (1,1)/Conbinational logic/PACK ==
  n0 : Inport
  n1 : Inport  Port=2
  n2 : Inport  Port=3
  n3 : Inport  Port=4
  n4 : Inport  Port=5
  n5 : Inport  Port=6
  n6 : Inport  Port=7
  n7 : Inport  Port=8
  Q : Inport  Port=9
  AND_Q_eq2 : Logic  AllPortsSameDT=off  OutDataTypeStr=boolean
  C2 : Constant  Value=2  OutDataTypeStr=fixdt(0,4,0)
  C3 : Constant  Value=3  OutDataTypeStr=fixdt(0,4,0)
  OR_E : Logic  Operator=OR  AllPortsSameDT=off  OutDataTypeStr=boolean
  Sum_N : Sum  Inputs=++++++++  AccumDataTypeStr=fixdt(0,4,0)  OutDataTypeStr=fixdt(0,4,0)
  eq2 : RelationalOperator  Operator===  OutDataTypeStr=boolean  RndMeth=Simplest  InputSameDT=off
  eq3 : RelationalOperator  Operator===  OutDataTypeStr=boolean  RndMeth=Simplest  InputSameDT=off
  E : Outport
  wires:
  Sum_N/1 -> eq2/1, eq3/1
  C3/1 -> eq3/2
  n7/1 -> Sum_N/8
  Q/1 -> AND_Q_eq2/1
  n0/1 -> Sum_N/1
  n3/1 -> Sum_N/4
  eq3/1 -> OR_E/1
  n1/1 -> Sum_N/2
  n4/1 -> Sum_N/5
  n2/1 -> Sum_N/3
  n6/1 -> Sum_N/7
  eq2/1 -> AND_Q_eq2/2
  C2/1 -> eq2/2
  OR_E/1 -> E/1
  AND_Q_eq2/1 -> OR_E/2
  n5/1 -> Sum_N/6

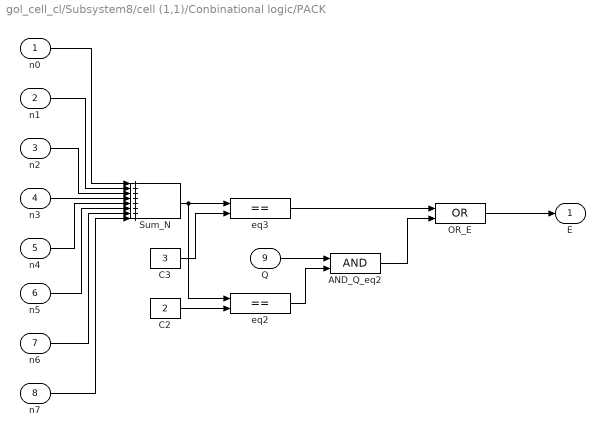
== system gol_cell_cl/Subsystem8/cell (1,1)/Conbinational logic/PACK ==
  n0 : Inport
  n1 : Inport  Port=2
  n2 : Inport  Port=3
  n3 : Inport  Port=4
  n4 : Inport  Port=5
  n5 : Inport  Port=6
  n6 : Inport  Port=7
  n7 : Inport  Port=8
  Q : Inport  Port=9
  AND_Q_eq2 : Logic  AllPortsSameDT=off  OutDataTypeStr=boolean
  C2 : Constant  Value=2  OutDataTypeStr=fixdt(0,4,0)
  C3 : Constant  Value=3  OutDataTypeStr=fixdt(0,4,0)
  OR_E : Logic  Operator=OR  AllPortsSameDT=off  OutDataTypeStr=boolean
  Sum_N : Sum  Inputs=++++++++  AccumDataTypeStr=fixdt(0,4,0)  OutDataTypeStr=fixdt(0,4,0)
  eq2 : RelationalOperator  Operator===  OutDataTypeStr=boolean  RndMeth=Simplest  InputSameDT=off
  eq3 : RelationalOperator  Operator===  OutDataTypeStr=boolean  RndMeth=Simplest  InputSameDT=off
  E : Outport
  wires:
  Sum_N/1 -> eq2/1, eq3/1
  C3/1 -> eq3/2
  n7/1 -> Sum_N/8
  Q/1 -> AND_Q_eq2/1
  n0/1 -> Sum_N/1
  n3/1 -> Sum_N/4
  eq3/1 -> OR_E/1
  n1/1 -> Sum_N/2
  n4/1 -> Sum_N/5
  n2/1 -> Sum_N/3
  n6/1 -> Sum_N/7
  eq2/1 -> AND_Q_eq2/2
  C2/1 -> eq2/2
  OR_E/1 -> E/1
  AND_Q_eq2/1 -> OR_E/2
  n5/1 -> Sum_N/6

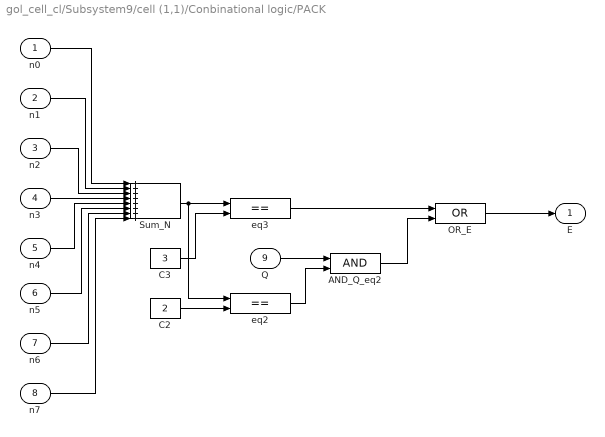
== system gol_cell_cl/Subsystem9/cell (1,1)/Conbinational logic/PACK ==
  n0 : Inport
  n1 : Inport  Port=2
  n2 : Inport  Port=3
  n3 : Inport  Port=4
  n4 : Inport  Port=5
  n5 : Inport  Port=6
  n6 : Inport  Port=7
  n7 : Inport  Port=8
  Q : Inport  Port=9
  AND_Q_eq2 : Logic  AllPortsSameDT=off  OutDataTypeStr=boolean
  C2 : Constant  Value=2  OutDataTypeStr=fixdt(0,4,0)
  C3 : Constant  Value=3  OutDataTypeStr=fixdt(0,4,0)
  OR_E : Logic  Operator=OR  AllPortsSameDT=off  OutDataTypeStr=boolean
  Sum_N : Sum  Inputs=++++++++  AccumDataTypeStr=fixdt(0,4,0)  OutDataTypeStr=fixdt(0,4,0)
  eq2 : RelationalOperator  Operator===  OutDataTypeStr=boolean  RndMeth=Simplest  InputSameDT=off
  eq3 : RelationalOperator  Operator===  OutDataTypeStr=boolean  RndMeth=Simplest  InputSameDT=off
  E : Outport
  wires:
  Sum_N/1 -> eq2/1, eq3/1
  C3/1 -> eq3/2
  n7/1 -> Sum_N/8
  Q/1 -> AND_Q_eq2/1
  n0/1 -> Sum_N/1
  n3/1 -> Sum_N/4
  eq3/1 -> OR_E/1
  n1/1 -> Sum_N/2
  n4/1 -> Sum_N/5
  n2/1 -> Sum_N/3
  n6/1 -> Sum_N/7
  eq2/1 -> AND_Q_eq2/2
  C2/1 -> eq2/2
  OR_E/1 -> E/1
  AND_Q_eq2/1 -> OR_E/2
  n5/1 -> Sum_N/6
